simulink model "PIDInvP"  (R2015b)
settings: Solver=ode4  StartTime=0.0  StopTime=10  FixedStep=.001  RelTol=1e-3
values from neighbouring files (symbols this model uses):
  xdistort = [1.4; -.7]    [PerformancePlots.m]
libraries: aerolibconvert2 x3, simulink x1
settings Model: Creator=Helene  LastModifiedBy=Helene

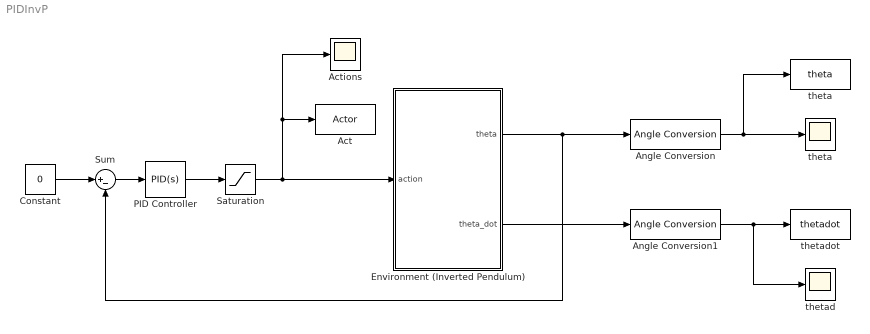
== system PIDInvP ==
  Act : ToWorkspace  VariableName=Actor  SaveFormat=Timeseries  SampleTime=-1
  Actions : Scope
  Angle Conversion : aerolibconvert2/Angle Conversion  IU=rad  OU=deg
  Angle Conversion1 : aerolibconvert2/Angle Conversion  IU=rad  OU=deg
  Constant : Constant  Value=0
  Environment (Inverted Pendulum) : Subsystem
  PID Controller : simulink/Continuous/PID Controller  Controller=PID  TimeDomain=Continuous-time  SampleTime=-1  IntegratorMethod=Forward Euler  FilterMethod=Forward Euler  Form=Parallel  UseFilter=on  ControllerParametersSource=internal  P=1.29854726716373  I=5.0615809805935  D=0.081803639155103  N=454.107025662928  InitialConditionSource=internal  InitialConditionForIntegrator=0  InitialConditionForFilter=0  ExternalReset=none  LimitOutput=off  UpperSaturationLimit=inf  LowerSaturationLimit=-inf  LinearizeAsGain=on  AntiWindupMode=none  Kb=1  TrackingMode=off  Kt=1  PParamMin=[]  PParamMax=[]  IParamMin=[]  IParamMax=[]  DParamMin=[]  DParamMax=[]  NParamMin=[]  NParamMax=[]  KbParamMin=[]  KbParamMax=[]  KtParamMin=[]  KtParamMax=[]  POutMin=[]  POutMax=[]  IOutMin=[]  IOutMax=[]  DOutMin=[]  DOutMax=[]  NOutMin=[]  NOutMax=[]  KbOutMin=[]  KbOutMax=[]  KtOutMin=[]  KtOutMax=[]  IntegratorOutMin=[]  IntegratorOutMax=[]  FilterOutMin=[]  FilterOutMax=[]  SumOutMin=[]  SumOutMax=[]  SumI1OutMin=[]  SumI1OutMax=[]  SumI2OutMin=[]  SumI2OutMax=[]  SumI3OutMin=[]  SumI3OutMax=[]  SumDOutMin=[]  SumDOutMax=[]  SaturationOutMin=[]  SaturationOutMax=[]  IntegratorContinuousStateAttributes=''  IntegratorStateMustResolveToSignalObject=off  IntegratorRTWStateStorageClass=Auto  FilterContinuousStateAttributes=''  FilterStateMustResolveToSignalObject=off  FilterRTWStateStorageClass=Auto  DifferentiatorICPrevScaledInput=0  DifferentiatorOutMin=[]  DifferentiatorOutMax=[]
  Saturation : Saturate  UpperLimit=0.1  LowerLimit=-0.1
  Sum : Sum  Inputs=|+-
  theta : Scope
  "theta " : ToWorkspace  VariableName=theta  SaveFormat=Timeseries  SampleTime=-1
  thetad : Scope
  thetadot : ToWorkspace  VariableName=thetadot  SaveFormat=Timeseries  SampleTime=-1
  wires:
  Angle Conversion/1 -> theta/1, "theta "/1
  PID Controller/1 -> Saturation/1
  Angle Conversion1/1 -> thetad/1, thetadot/1
  Environment (Inverted Pendulum)/2(theta_dot) -> Angle Conversion1/1
  Sum/1 -> PID Controller/1
  Constant/1 -> Sum/1
  Saturation/1 -> Environment (Inverted Pendulum)/1(action), Actions/1, Act/1
  Environment (Inverted Pendulum)/1(theta) -> Angle Conversion/1, Sum/2

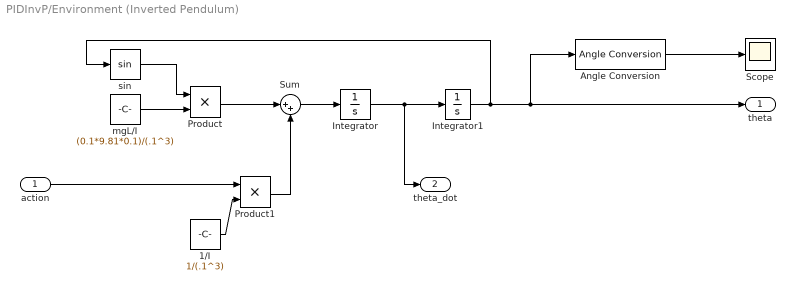
== system PIDInvP/Environment (Inverted Pendulum) ==
  action : Inport
  1/I : Constant  Value=1/(.1^3)
  Angle Conversion : aerolibconvert2/Angle Conversion  IU=rad  OU=deg
  Integrator : Integrator
  Integrator1 : Integrator  InitialCondition=xdistort
  Product : Product
  Product1 : Product
  Scope : Scope
  Sum : Sum  Inputs=|++
  mgL/I : Constant  Value=(0.1*9.81*0.1)/(.1^3)
  sin : Trigonometry
  theta : Outport
  theta_dot : Outport  Port=2
  wires:
  Integrator/1 -> theta_dot/1, Integrator1/1
  action/1 -> Product1/1
  mgL/I/1 -> Product/2
  Product/1 -> Sum/1
  Sum/1 -> Integrator/1
  sin/1 -> Product/1
  1/I/1 -> Product1/2
  Product1/1 -> Sum/2
  Angle Conversion/1 -> Scope/1
  Integrator1/1 -> theta/1, Angle Conversion/1, sin/1
